simulink model "Problem_9"  (R2020a)
settings: Solver=VariableStepAuto  StartTime=0.0  StopTime=10.0  RelTol=1e-3
values from neighbouring files (symbols this model uses):
  Ke = 0.06902    [Problem_9_mfile.m]
  taue = 151.51*10^-6    (= 0.00015151)    [Problem_9_mfile.m]
  taum = 0.0161    [Problem_9_mfile.m]
settings Model: Creator=Saqlain  LastModifiedBy=Saqlain

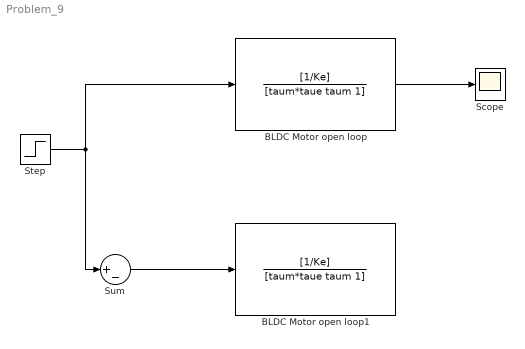
== system Problem_9 ==
  BLDC Motor open loop : TransferFcn  Numerator=[1/Ke]  Denominator=[taum*taue taum 1]
  BLDC Motor open loop1 : TransferFcn  Numerator=[1/Ke]  Denominator=[taum*taue taum 1]
  Scope : Scope
  Step : Step  SampleTime=0
  Sum : Sum  Inputs=|+-
  wires:
  Step/1 -> Sum/1, BLDC Motor open loop/1
  BLDC Motor open loop/1 -> Scope/1
  Sum/1 -> BLDC Motor open loop1/1
